simulink model "FIR_floating"  (R2017a)
settings: Solver=VariableStepAuto  StartTime=0.0  StopTime=10.0  RelTol=1e-3
settings Model: Creator=Arthur  LastModifiedBy=Arthur

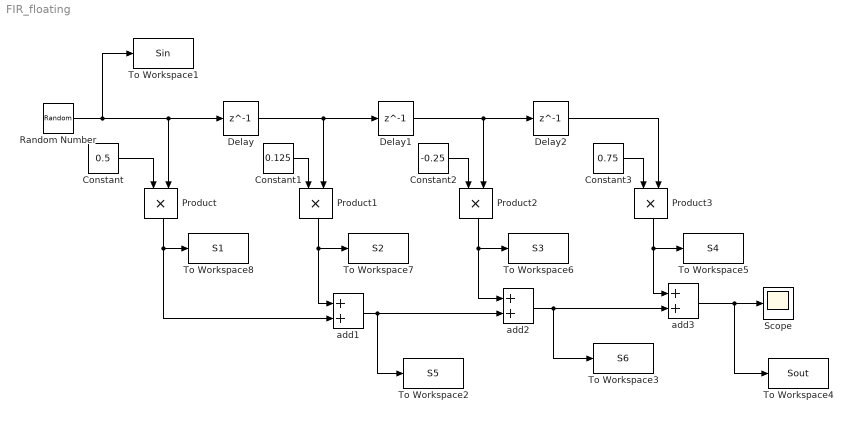
== system FIR_floating ==
  Constant : Constant  Value=0.5
  Constant1 : Constant  Value=0.125
  Constant2 : Constant  Value=-0.25
  Constant3 : Constant  Value=0.75
  Delay : Delay  DelayLength=1
  Delay1 : Delay  DelayLength=1
  Delay2 : Delay  DelayLength=1
  Product{,1..3} (4 alike) : Product
  Random Number : RandomNumber  SampleTime=0.1
  Scope : Scope
  To Workspace1 : ToWorkspace  VariableName=Sin  SampleTime=-1
  To Workspace2 : ToWorkspace  VariableName=S5  SampleTime=-1
  To Workspace3 : ToWorkspace  VariableName=S6  SampleTime=-1
  To Workspace4 : ToWorkspace  VariableName=Sout  SampleTime=-1
  To Workspace5 : ToWorkspace  VariableName=S4  SampleTime=-1
  To Workspace6 : ToWorkspace  VariableName=S3  SampleTime=-1
  To Workspace7 : ToWorkspace  VariableName=S2  SampleTime=-1
  To Workspace8 : ToWorkspace  VariableName=S1  SampleTime=-1
  add1 : Sum
  add2 : Sum
  add3 : Sum
  wires:
  Random Number/1 -> To Workspace1/1, Product/2, Delay/1
  Delay/1 -> Product1/2, Delay1/1
  Delay1/1 -> Product2/2, Delay2/1
  add3/1 -> To Workspace4/1, Scope/1
  Product3/1 -> To Workspace5/1, add3/1
  Constant/1 -> Product/1
  Constant1/1 -> Product1/1
  Constant2/1 -> Product2/1
  Constant3/1 -> Product3/1
  Delay2/1 -> Product3/2
  add2/1 -> To Workspace3/1, add3/2
  Product2/1 -> To Workspace6/1, add2/1
  add1/1 -> To Workspace2/1, add2/2
  Product1/1 -> To Workspace7/1, add1/1
  Product/1 -> To Workspace8/1, add1/2
